simulink model "pseudorandom"  (R2015a)
settings: Solver=ode45  StartTime=0.0  StopTime=10.0  RelTol=1e-3
libraries: PoliArd x6, simulink x1
settings Model: CovModelRefEnable=off  Creator=gsavaia  LastModifiedBy=gsavaia
settings DataIOCC: SaveFormat=Dataset
settings HardwareCC: ProdBitPerPointer=64  ProdLargestAtomicFloat=Float  ProdIntDivRoundTo=Zero  ProdEndianess=LittleEndian  ProdHWDeviceType=Specified
settings GRTTargetCC: GeneratePreprocessorConditionals=Use local settings

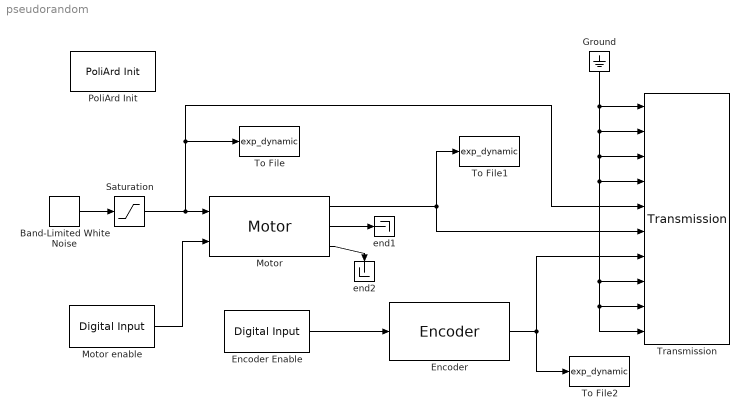
== system pseudorandom ==
  Band-Limited White Noise : simulink/Sources/Band-Limited White Noise  Cov=[0.1]  Ts=0.1  seed=[61292]
  Encoder : PoliArd/Encoder  EncoderID=1  dt_enc=-1
  Encoder Enable : PoliArd/Digital Input  DI_pin=2  DIsample=-1
  Ground : Ground
  Motor : PoliArd/Motor  MotorID=1  DC_bus_mask=12  dt_mot=-1
  Motor enable : PoliArd/Digital Input  DI_pin=3  DIsample=-1
  PoliArd Init : PoliArd/PoliArd Init
  Saturation : Saturate  UpperLimit=4  LowerLimit=-4
  To File : ToFile  Filename=exp_dynamic  MatrixName=v
  To File1 : ToFile  Filename=exp_dynamic  MatrixName=i
  To File2 : ToFile  Filename=exp_dynamic  MatrixName=d
  Transmission : PoliArd/Transmission  sample_freq=100  sig_to_send=6
  end1 : Terminator
  end2 : Terminator
  wires:
  Motor enable/1 -> Motor/2
  Ground/1 -> Transmission/10, Transmission/9, Transmission/8, Transmission/4, Transmission/3, Transmission/2, Transmission/1
  Encoder/1 -> Transmission/7, To File2/1
  Encoder Enable/1 -> Encoder/1
  Motor/2 -> end1/1
  Motor/3 -> end2/1
  Motor/1 -> To File1/1, Transmission/6
  Band-Limited White Noise/1 -> Saturation/1
  Saturation/1 -> To File/1, Transmission/5, Motor/1
